simulink model "sim_quadrotor_test"  (R2018a)
settings: Solver=ode45  StartTime=0.0  StopTime=1  RelTol=1e-3  EnableMultiTasking=on
libraries: slident x1
settings Model: Creator=rblan  LastModifiedBy=rblan
settings DataIOCC: LimitDataPoints=on  SaveFormat=Array
settings OptimizationCC: LifeSpan=inf
settings DebuggingCC: SFUnexpectedBacktrackingDiag=warning  SFNoUnconditionalDefaultTransitionDiag=warning  SFExecutionAtInitializationDiag=none
settings HardwareCC: ProdBitPerPointer=32  ProdBitPerSizeT=32  ProdBitPerPtrDiffT=32  ProdLargestAtomicFloat=None  ProdIntDivRoundTo=Undefined  ProdEndianess=Unspecified  ProdWordSize=32  ProdHWDeviceType=32-bit Generic
settings ModelReferenceCC: PropagateSignalLabelsOutOfModel=off
settings CodeAppCC: StateflowObjectComments=on
settings GRTTargetCC: TargetLangStandard=C89/C90 (ANSI)  GeneratePreprocessorConditionals=Disable all
settings ConfigComp: CovMetricSettings=dw  CovHtmlReporting=on  CovSaveCumulativeToWorkspaceVar=on  CovSaveSingleToWorkspaceVar=on  CovExternalEMLEnable=off

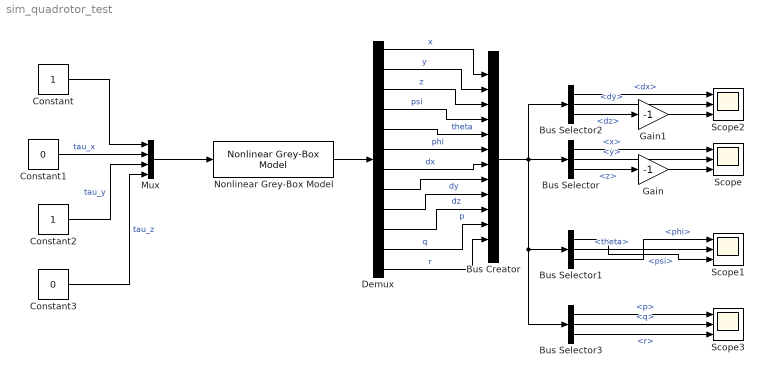
== system sim_quadrotor_test ==
  Bus Creator : BusCreator  Inputs=12
  Bus Selector : BusSelector  OutputSignals=x,y,z
  Bus Selector1 : BusSelector  OutputSignals=psi,theta,phi
  Bus Selector2 : BusSelector  OutputSignals=dx,dy,dz
  Bus Selector3 : BusSelector  OutputSignals=p,q,r
  Constant : Constant
  Constant1 : Constant  Value=0
  Constant2 : Constant
  Constant3 : Constant  Value=0
  Demux : Demux  Outputs=12
  Gain : Gain  Gain=-1
  Gain1 : Gain  Gain=-1
  Mux : Mux
  Nonlinear Grey-Box Model : slident/Models/Nonlinear Grey-Box Model  nlsys=quadrotor_m  X0='m'
      settings: SourceProductName=System Identification Toolbox  SourceProductBaseCode=ID
  Scope{,1..3} (4 alike) : Scope  NumInputPorts=3
  wires:
  Nonlinear Grey-Box Model/1 -> Demux/1
  Demux/1 -> Bus Creator/1  "x"
  Demux/2 -> Bus Creator/2  "y"
  Demux/3 -> Bus Creator/3  "z"
  Demux/4 -> Bus Creator/4  "psi"
  Demux/5 -> Bus Creator/5  "theta"
  Demux/6 -> Bus Creator/6  "phi"
  Demux/7 -> Bus Creator/7  "dx"
  Demux/8 -> Bus Creator/8  "dy"
  Demux/9 -> Bus Creator/9  "dz"
  Demux/10 -> Bus Creator/10  "p"
  Demux/11 -> Bus Creator/11  "q"
  Demux/12 -> Bus Creator/12  "r"
  Bus Selector/1 -> Scope/1  "<x>"
  Bus Selector/2 -> Scope/2  "<y>"
  Bus Selector/3 -> Gain/1  "<z>"
  Bus Selector1/2 -> Scope1/2  "<theta>"
  Mux/1 -> Nonlinear Grey-Box Model/1
  Constant/1 -> Mux/1
  Constant1/1 -> Mux/2  "tau_x"
  Constant2/1 -> Mux/3  "tau_y"
  Constant3/1 -> Mux/4  "tau_z"
  Bus Selector1/3 -> Scope1/1  "<phi>"
  Bus Selector1/1 -> Scope1/3  "<psi>"
  Bus Selector2/1 -> Scope2/1  "<dx>"
  Bus Selector2/2 -> Scope2/2  "<dy>"
  Bus Selector2/3 -> Gain1/1  "<dz>"
  Bus Selector3/1 -> Scope3/1  "<p>"
  Bus Selector3/2 -> Scope3/2  "<q>"
  Bus Selector3/3 -> Scope3/3  "<r>"
  Bus Creator/1 -> Bus Selector2/1, Bus Selector3/1, Bus Selector1/1, Bus Selector/1
  Gain/1 -> Scope/3
  Gain1/1 -> Scope2/3
